simulink model "PID_enable_ROS2020b"  (R2020b)
settings: Solver=FixedStepAuto  StartTime=0.0  StopTime=inf  FixedStep=1/120  RelTol=1e-3
undefined symbols (not defined in the file): DiscIntNeverNeededParam, Flm, Frm, Jx_ref, Jy_ref, Jz_ref, m_ref, pos_ref, psi_ref, psidot_ref, Rlm, Rrm, t_ref, vel_ref, Yaw
libraries: robotlib x3, simulink x2, dspfdesign x1, aerolibanimutils x1
settings Model: Creator=iris  LastModifiedBy=iris
settings OptimizationCC: EnhancedBackFolding=on  PassReuseOutputArgsAs=Individual arguments  ZeroExternalMemoryAtStartup=off  ZeroInternalMemoryAtStartup=off  MaxStackSize=64  OptimizeBlockOrder=speed  DifferentSizesBufferReuse=on  OptimizationCustomize=off  EfficientTunableParamExpr=on
settings DebuggingCC: ParameterTunabilityLossMsg=error  SFMachineParentedDataDiag=error
settings HardwareCC: ProdBitPerPointer=32  ProdBitPerSizeT=32  ProdBitPerPtrDiffT=32  ProdLargestAtomicFloat=None  ProdIntDivRoundTo=Undefined  ProdEndianess=Unspecified  ProdWordSize=32  ProdHWDeviceType=Generic->Unspecified (assume 32-bit Generic)
settings SFSimCC: MATLABDynamicMemAlloc=off  SimTargetLang=C++
settings RTWCC: Description=Embedded Coder  SystemTargetFile=ert.tlc  HardwareBoard=Robot Operating System (ROS)  TLCOptions="-aInlineSetEventsForThisBaseRateFcn=TLC_FALSE -aSuppressMultiTaskScheduler=TLC_FALSE  -aRateBasedStepFcn=0"  TemplateMakefile=ert_default_tmf  Toolchain=Catkin  TargetLang=C++
settings CodeAppCC: ForceParamTrailComments=on  IgnoreCustomStorageClasses=off  OperatorAnnotations=on  SimulinkDataObjDesc=on  SFDataObjDesc=on  InsertBlockDesc=on
settings ERTTargetCC: SupportVariableSizeSignals=on

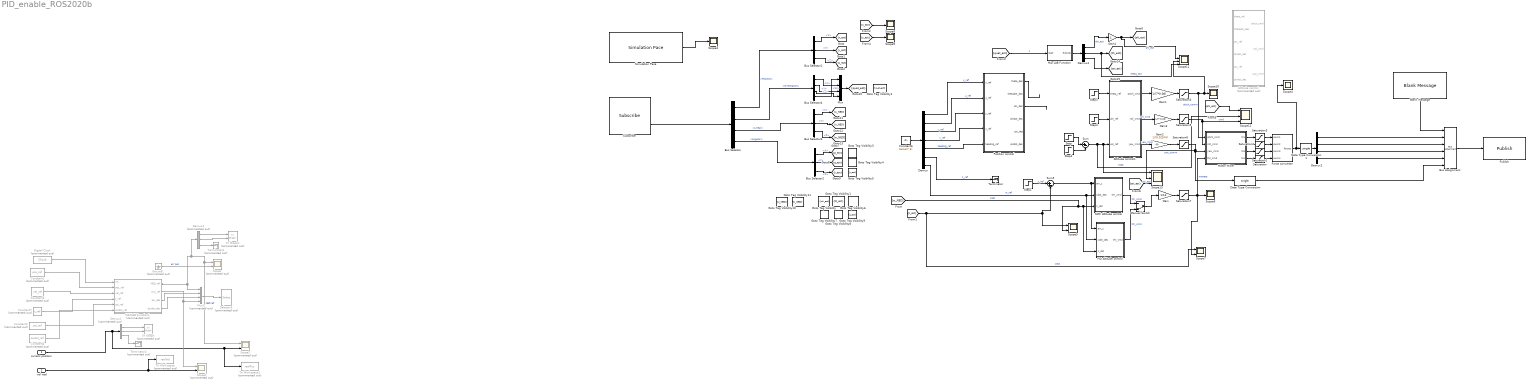
== system PID_enable_ROS2020b ==
  current position : Inport
  vel ned : Inport  Port=2
  Attitude control : Subsystem  Commented=on
  Attitude control1 : Subsystem
  Blank Message : robotlib/Blank Message  messageClass=Message  entityType=robotics_demo/QuadForce  messageType=robotics_demo/QuadForce  SampleTime=inf  legacyBusStruct=off
  Bus Assignment : BusAssignment  AssignedSignals=Frm,Rlm,Flm,Rrm,Yaw
  Bus Selector : BusSelector  OutputSignals=Pose.Pose.Position,Pose.Pose.Orientation,Twist.Twist.Linear,Twist.Twist.Angular
  Bus Selector1 : BusSelector  OutputSignals=X,Y,Z
  Bus Selector2 : BusSelector  OutputSignals=X,Y,Z
  Bus Selector3 : BusSelector  OutputSignals=X,Y,Z
  Bus Selector4 : BusSelector  OutputSignals=X,Y,Z,W
  Constant1 : Constant  Commented=on  Value=pos_ref
  Constant2 : Constant  Commented=on  Value=psi_ref
  Constant3 : Constant  Commented=on  Value=vel_ref
  Constant4 : Constant  Commented=on  Value=psidot_ref
  Constant5 : Constant  Commented=on  Value=t_ref
  Constant6 : Constant  Value=zeros(7,1)
  Data Type Conversion : DataTypeConversion  OutDataTypeStr=single
  Data Type Conversion1 : DataTypeConversion  OutDataTypeStr=single
  Demux : Demux  Outputs=7
  Demux1 : Demux  Commented=on  Outputs=3
  Demux2 : Demux
  Demux3 : Demux  Commented=on  Outputs=3
  Demux4 : Demux  Outputs=3
  Digital Clock : DigitalClock  Commented=on  SampleTime=-1
  Force converter : MATLAB Function  TreatAsAtomicUnit=on
  Gain : Gain  Gain=1/14
  Gain1 : Gain  Gain=1/(7*0.08)
  Gain2 : Gain  Gain=1/(0.025*4)
  Gain3 : Gain  Gain=1/(7*0.08)
  Gain4 : Gain
  Goto Tag Visibility : GotoTagVisibility  GotoTag=phi_est
  Goto Tag Visibility1 : GotoTagVisibility  GotoTag=th_est
  Goto Tag Visibility10 : GotoTagVisibility  GotoTag=u_NED
  Goto Tag Visibility11 : GotoTagVisibility  GotoTag=v_NED
  Goto Tag Visibility2 : GotoTagVisibility  GotoTag=quat_est
  Goto Tag Visibility3 : GotoTagVisibility  GotoTag=p_est
  Goto Tag Visibility4 : GotoTagVisibility  GotoTag=q_est
  Goto Tag Visibility5 : GotoTagVisibility  GotoTag=r_est
  Goto Tag Visibility6 : GotoTagVisibility  GotoTag=psi_est
  Goto Tag Visibility7 : GotoTagVisibility  GotoTag=x_est
  Goto Tag Visibility8 : GotoTagVisibility  GotoTag=y_est
  Goto Tag Visibility9 : GotoTagVisibility  GotoTag=z_est
  Ground1 : Ground  Commented=on
  MATLAB Function : MATLAB Function  TreatAsAtomicUnit=on
  MATLAB Function1 : MATLAB Function  Commented=on  TreatAsAtomicUnit=on
  Manual Switch : ManualSwitch  CurrentSetting=0
  Motor Mixer : MATLAB Function  TreatAsAtomicUnit=on
  Mux : Mux
  Mux1 : Mux  Commented=on
  PID Altitude control : Subsystem
  Position control : Subsystem
  Publish : robotlib/Publish  topicSource=Specify your own  topic=/motorForce  messageType=robotics_demo/QuadForce  legacyBusStruct=off  messageQueueLength=1
  SMC Altitude control : Subsystem
  Saturation : Saturate  UpperLimit=2000  LowerLimit=0
  Saturation1 : Saturate  UpperLimit=2000  LowerLimit=0
  Saturation2 : Saturate  UpperLimit=2000  LowerLimit=0
  Saturation3 : Saturate  UpperLimit=2000  LowerLimit=1000
  Saturation4 : Saturate  UpperLimit=1  LowerLimit=-1
  Saturation5 : Saturate  UpperLimit=1  LowerLimit=-1
  Saturation6 : Saturate  UpperLimit=1  LowerLimit=-1
  Saturation7 : Saturate  UpperLimit=1  LowerLimit=0
  Scope : Scope  Commented=on  NumInputPorts=2
  Scope1 : Scope  Commented=on  NumInputPorts=2
  Scope{3..4,6,8..10} (6 alike) : Scope
  Scope11 : Scope  NumInputPorts=4
  Scope12 : Scope  NumInputPorts=3
  Scope13 : Scope  NumInputPorts=3
  Scope2 : Scope  Commented=on  NumInputPorts=2
  Scope5 : Scope  NumInputPorts=2
  Scope7 : Scope  NumInputPorts=2
  Selector3 : Selector  Commented=on  InputPortWidth=8  IndexOptions=Index vector (dialog)  Indices=[1 6 2 7 4 3 8]  OutputSizes=1
  Simulation Pace : aerolibanimutils/Simulation Pace  SimulationPace=1  SleepMode=Auto  OutputPaceError=on  SampleTime=1/30
  Step : Step  Time=6  After=10/180*pi  SampleTime=0
  Step1 : Step  After=10
  Step2 : Step  Time=7  After=10/180*pi  SampleTime=0
  Step3 : Step  Time=0  After=0  SampleTime=0
  Step4 : Step  Time=0  After=0  SampleTime=0
  Subscribe : robotlib/Subscribe  topicSource=Specify your own  topic=/odom  messageType=nav_msgs/Odometry  SampleTime=-1  legacyBusStruct=off  messageQueueLength=1
  Sum : Sum  Inputs=|+-
  Sum5 : Sum  Inputs=|+-
  Terminator : Terminator
  Terminator2 : Terminator  Commented=on
  Terminator3 : Terminator  Commented=on
  To Workspace : ToWorkspace  Commented=on  VariableName=realVel  SaveFormat=Timeseries  SampleTime=-1
  To Workspace1 : ToWorkspace  Commented=on  VariableName=realPos  SaveFormat=Timeseries  SampleTime=-1
  XY Graph : simulink/Sinks/XY Graph  Commented=on  xmin=-20  xmax=20  ymin=-20  ymax=20  st=-1
  XY Graph1 : simulink/Sinks/XY Graph  Commented=on  xmin=-20  xmax=20  ymin=-20  ymax=20  st=-1
  tag scope: p_est=scoped, phi_est=scoped, psi_est=scoped, q_est=scoped, quat_est=scoped, r_est=scoped, th_est=scoped, u_NED=scoped, v_NED=scoped, x_est=scoped, y_est=scoped, z_est=scoped
  wires:
  Demux1/1 -> XY Graph/1
  current position/1 -> To Workspace1/1, Scope2/2, Demux1/1
  Demux3/3 -> Terminator3/1
  Demux3/2 -> XY Graph1/2
  Constant2/1 -> MATLAB Function1/5(psi_ref)
  MATLAB Function1/3(psi_des) -> Mux1/2
  Demux1/2 -> XY Graph/2
  Mux1/1 -> Selector3/1
  Constant3/1 -> MATLAB Function1/3(vel_ref)
  MATLAB Function1/2(uvw_ref) -> Scope1/1, Mux1/4
  Constant1/1 -> MATLAB Function1/2(pos_ref)
  Ground1/1 -> Scope/2  "err pos"
  vel ned/1 -> To Workspace/1, Scope1/2
  MATLAB Function1/1(NED_ref) -> Mux1/1, Demux3/1, Scope2/1, Scope/1  "NED ref"
  Constant5/1 -> MATLAB Function1/4(t_ref)
  Demux3/1 -> XY Graph1/1
  Digital Clock/1 -> MATLAB Function1/1(clk)
  MATLAB Function1/4(psidot_des) -> Mux1/3
  Demux1/3 -> Terminator2/1
  Constant4/1 -> MATLAB Function1/6(psidot_ref)
  Motor Mixer/3(M3) -> Saturation1/1
  Demux4/1 -> Gain4/1  "phi_est"
  SMC Altitude control/1(thr_cmd) -> Manual Switch/1  "thr_cmd"
  Demux4/2 -> [th_est], Scope11/4  "theta_est"
  Saturation2/1 -> Force converter/2(pwm2)
  Bus Selector/1 -> Bus Selector1/1  "<Position>"
  Bus Selector3/1 -> [u_NED]  "<X>"
  Demux/6 -> Terminator/1  "z_ref"
  Demux/7 -> PID Altitude control/2(zdot_des), SMC Altitude control/2(zdot_des)  "w_ref"
  Demux/2 -> Position control/2(u_ref)  "u_ref"
  Saturation/1 -> Force converter/4(pwm4)
  PID Altitude control/1(thr_cmd) -> Manual Switch/2  "thr_cmd"
  Bus Selector/2 -> Bus Selector4/1  "<Orientation>"
  Attitude control1/1(pitch_cmd) -> Gain1/1
  Bus Selector2/3 -> [r_est]  "<Z>"
  [w_NED] -> PID Altitude control/3(z_dot), SMC Altitude control/3(z_dot), Scope5/2  "zdot"
  Gain1/1 -> Saturation4/1
  [quat_est] -> MATLAB Function/1(quat)  "z"
  Demux/5 -> Position control/5(heading_ref)  "heading_ref"
  Gain3/1 -> Saturation5/1
  Demux/3 -> Position control/3(y_ref)  "y_ref"
  Bus Selector1/3 -> [z_est]  "<Z>"
  Saturation3/1 -> Force converter/1(pwm1)
  Subscribe/2 -> Bus Selector/1
  Gain/1 -> Saturation7/1
  Sum5/1 -> PID Altitude control/1(err_z), SMC Altitude control/1(err_z)
  Bus Selector4/2 -> Mux/3  "<Y>"
  Manual Switch/1 -> Gain/1
  Bus Selector4/3 -> Mux/4  "<Z>"
  Motor Mixer/1(M1) -> Saturation3/1
  Bus Selector/4 -> Bus Selector2/1  "<Angular>"
  Bus Selector3/3 -> [w_NED]  "<Z>"
  Gain2/1 -> Saturation6/1
  Constant6/1 -> Demux/1
  Bus Selector4/1 -> Mux/2  "<X>"
  Bus Assignment/1 -> Publish/1
  Mux/1 -> [quat_est]
  Blank Message/1 -> Bus Assignment/1
  Force converter/1(forces) -> Scope4/1, Data Type Conversion1/1
  Saturation1/1 -> Force converter/3(pwm3)
  Attitude control1/2(roll_cmd) -> Gain3/1  "roll_cmd"
  Bus Selector2/1 -> [p_est]  "<X>"
  Attitude control1/3(yaw_cmd) -> Gain2/1  "yaw_cmd"
  Step1/1 -> Sum5/1  "z_ref"
  Saturation7/1 -> Scope7/2, Motor Mixer/4(thr_cmd), Scope6/1  "maneta"
  Bus Selector1/2 -> [y_est]  "<Y>"
  Data Type Conversion/1 -> Bus Assignment/6
  Demux4/3 -> [psi_est]
  MATLAB Function/1(eulAng) -> Demux4/1
  Bus Selector/3 -> Bus Selector3/1  "<Linear>"
  Data Type Conversion1/1 -> Demux2/1
  Bus Selector1/1 -> [x_est]  "<X>"
  [z_est] -> Scope7/1, Scope5/1, Sum5/2  "zest"
  Motor Mixer/2(M2) -> Saturation2/1
  Bus Selector2/2 -> [q_est]  "<Y>"
  Demux/4 -> Position control/4(v_ref)  "v_ref"
  Demux/1 -> Position control/1(x_ref)  "x_ref"
  Saturation4/1 -> Motor Mixer/1(pitch_cmd), Scope11/3, Scope10/1  "pitch_comm"
  Motor Mixer/4(M4) -> Saturation/1
  Bus Selector3/2 -> [v_NED]  "<Y>"
  Simulation Pace/1 -> Scope3/1
  Step/1 -> Sum/1
  Sum/1 -> Attitude control1/3(psi_ref), Scope13/1, Scope12/2  "step"
  Step2/1 -> Sum/2
  [y_est] -> Scope9/1
  [x_est] -> Scope8/1
  Saturation5/1 -> Motor Mixer/2(roll_cmd), Scope12/3  "cmd"
  Demux2/1 -> Bus Assignment/2
  Demux2/2 -> Bus Assignment/3
  Demux2/4 -> Bus Assignment/5
  Demux2/3 -> Bus Assignment/4
  Bus Selector4/4 -> Mux/1  "<W>"
  Gain4/1 -> [phi_est], Scope11/2  "phi_est"
  [phi_est] -> Scope12/1
  Saturation6/1 -> Scope13/2, Data Type Conversion/1, Motor Mixer/3(yaw_cmd)  "yaw_comm"
  [psi_est] -> Scope13/3  "psi_est"
  Position control/1(theta_des) -> ?
  Position control/3(phi_des) -> ?
  Step3/1 -> Attitude control1/1(theta_ref)
  Step4/1 -> Attitude control1/2(phi_ref)

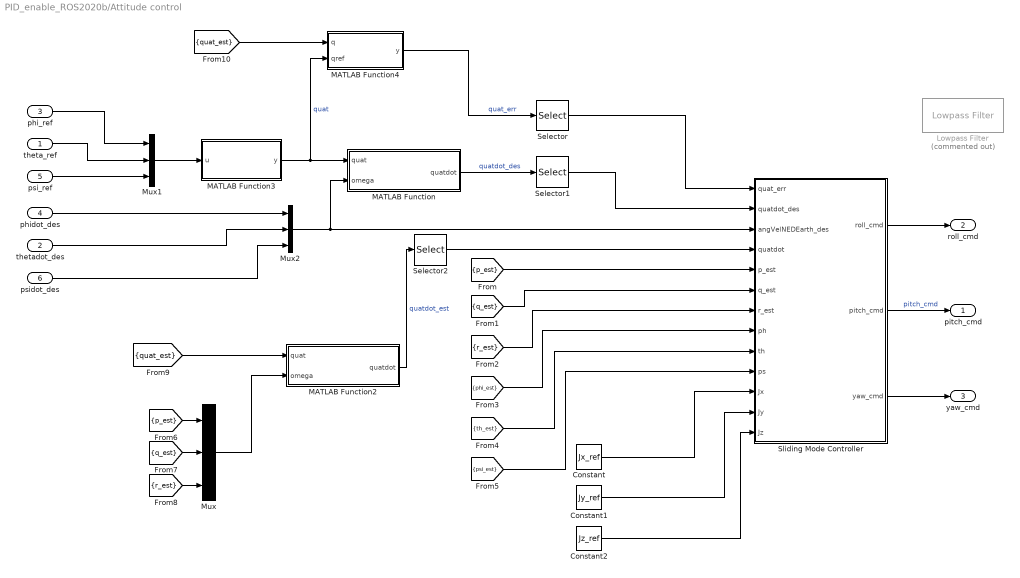
== system PID_enable_ROS2020b/Attitude control ==
  theta_ref : Inport
  thetadot_des : Inport  Port=2
  phi_ref : Inport  Port=3
  phidot_des : Inport  Port=4
  psi_ref : Inport  Port=5
  psidot_des : Inport  Port=6
  Constant : Constant  Value=Jx_ref
  Constant1 : Constant  Value=Jy_ref
  Constant2 : Constant  Value=Jz_ref
  Lowpass Filter : dspfdesign/Lowpass Filter  Commented=on  FilterType=FIR  DesignForMinimumOrder=on  FilterOrder=50  PassbandFrequency=100  StopbandFrequency=1000  PassbandRipple=0.1  StopbandAttenuation=40  InheritSampleRate=off  SampleRate=44100  SimulateUsing=Interpreted execution  roundingMode=Floor  coeffsDataTypeStr=fixdt(1,16)
  MATLAB Function : MATLAB Function  TreatAsAtomicUnit=on
  MATLAB Function2 : MATLAB Function  TreatAsAtomicUnit=on
  MATLAB Function3 : MATLAB Function  TreatAsAtomicUnit=on
  MATLAB Function4 : MATLAB Function  TreatAsAtomicUnit=on
  Mux : Mux  Inputs=3
  Mux1 : Mux  Inputs=3
  Mux2 : Mux  Inputs=3
  Selector : Selector  InputPortWidth=4  IndexOptions=Index vector (dialog)  Indices=[2:4]  OutputSizes=1
  Selector1 : Selector  InputPortWidth=4  IndexOptions=Index vector (dialog)  Indices=[2:4]  OutputSizes=1
  Selector2 : Selector  InputPortWidth=4  IndexOptions=Index vector (dialog)  Indices=[2:4]  OutputSizes=1
  Sliding Mode Controller : MATLAB Function  TreatAsAtomicUnit=on
  pitch_cmd : Outport  VectorParamsAs1DForOutWhenUnconnected=off
  roll_cmd : Outport  Port=2  VectorParamsAs1DForOutWhenUnconnected=off
  yaw_cmd : Outport  Port=3  VectorParamsAs1DForOutWhenUnconnected=off
  wires:
  [quat_est] -> MATLAB Function2/1(quat)
  MATLAB Function4/1(y) -> Selector/1  "quat_err"
  Mux1/1 -> MATLAB Function3/1(u)
  [r_est] -> Mux/3
  thetadot_des/1 -> Mux2/2
  [phi_est] -> Sliding Mode Controller/8(ph)
  [q_est] -> Mux/2
  Selector1/1 -> Sliding Mode Controller/2(quatdot_des)
  MATLAB Function2/1(quatdot) -> Selector2/1  "quatdot_est"
  [psi_est] -> Sliding Mode Controller/10(ps)
  Mux2/1 -> MATLAB Function/2(omega), Sliding Mode Controller/3(angVelNEDEarth_des)
  Selector/1 -> Sliding Mode Controller/1(quat_err)
  MATLAB Function/1(quatdot) -> Selector1/1  "quatdot_des"
  Mux/1 -> MATLAB Function2/2(omega)
  [q_est] -> Sliding Mode Controller/6(q_est)
  MATLAB Function3/1(y) -> MATLAB Function4/2(qref), MATLAB Function/1(quat)  "quat"
  [p_est] -> Sliding Mode Controller/5(p_est)
  Constant2/1 -> Sliding Mode Controller/13(Jz)
  Constant1/1 -> Sliding Mode Controller/12(Jy)
  [r_est] -> Sliding Mode Controller/7(r_est)
  Selector2/1 -> Sliding Mode Controller/4(quatdot)
  [th_est] -> Sliding Mode Controller/9(th)
  [p_est] -> Mux/1
  Sliding Mode Controller/2(pitch_cmd) -> pitch_cmd/1  "pitch_cmd"
  Constant/1 -> Sliding Mode Controller/11(Jx)
  theta_ref/1 -> Mux1/2
  phi_ref/1 -> Mux1/1
  psi_ref/1 -> Mux1/3
  [quat_est] -> MATLAB Function4/1(q)
  phidot_des/1 -> Mux2/1
  psidot_des/1 -> Mux2/3
  Sliding Mode Controller/1(roll_cmd) -> roll_cmd/1
  Sliding Mode Controller/3(yaw_cmd) -> yaw_cmd/1

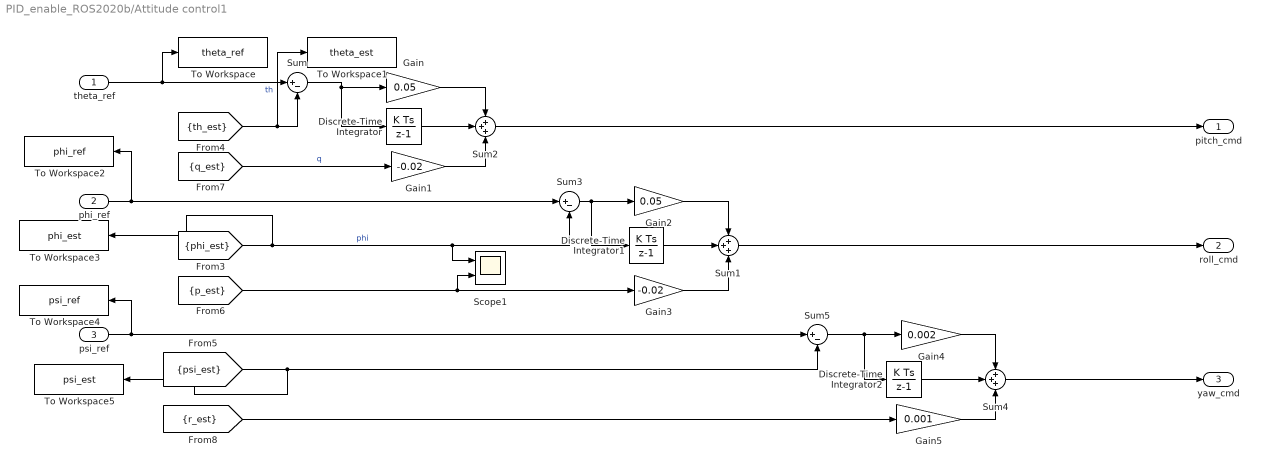
== system PID_enable_ROS2020b/Attitude control1 ==
  theta_ref : Inport
  phi_ref : Inport  Port=2
  psi_ref : Inport  Port=3
  Discrete-Time Integrator : DiscreteIntegrator  gainval=0.001  SampleTime=-1  ICPrevOutput=DiscIntNeverNeededParam  ICPrevScaledInput=DiscIntNeverNeededParam
  Discrete-Time Integrator1 : DiscreteIntegrator  gainval=0.001  SampleTime=-1  ICPrevOutput=DiscIntNeverNeededParam  ICPrevScaledInput=DiscIntNeverNeededParam
  Discrete-Time Integrator2 : DiscreteIntegrator  gainval=0.001  SampleTime=-1  UpperSaturationLimit=0.2  LowerSaturationLimit=-0.2  ICPrevOutput=DiscIntNeverNeededParam  ICPrevScaledInput=DiscIntNeverNeededParam
  Gain : Gain  Gain=0.05
  Gain1 : Gain  Gain=-0.02
  Gain2 : Gain  Gain=0.05
  Gain3 : Gain  Gain=-0.02
  Gain4 : Gain  Gain=0.002
  Gain5 : Gain  Gain=0.001
  Scope1 : Scope  NumInputPorts=2
  Sum : Sum  Inputs=|+-
  Sum1 : Sum  Inputs=+++
  Sum2 : Sum  Inputs=+++
  Sum3 : Sum  Inputs=|+-
  Sum4 : Sum  Inputs=+++
  Sum5 : Sum  Inputs=|+-
  To Workspace : ToWorkspace  VariableName=theta_ref  SampleTime=-1
      settings: Save2DSignal=2-D array (concatenate along first dimension)
  To Workspace1 : ToWorkspace  VariableName=theta_est  SampleTime=-1
      settings: Save2DSignal=2-D array (concatenate along first dimension)
  To Workspace2 : ToWorkspace  VariableName=phi_ref  SampleTime=-1
      settings: Save2DSignal=2-D array (concatenate along first dimension)
  To Workspace3 : ToWorkspace  VariableName=phi_est  SampleTime=-1
      settings: Save2DSignal=2-D array (concatenate along first dimension)
  To Workspace4 : ToWorkspace  VariableName=psi_ref  SampleTime=-1
      settings: Save2DSignal=2-D array (concatenate along first dimension)
  To Workspace5 : ToWorkspace  VariableName=psi_est  SampleTime=-1
      settings: Save2DSignal=2-D array (concatenate along first dimension)
  pitch_cmd : Outport  VectorParamsAs1DForOutWhenUnconnected=off
  roll_cmd : Outport  Port=2  VectorParamsAs1DForOutWhenUnconnected=off
  yaw_cmd : Outport  Port=3  VectorParamsAs1DForOutWhenUnconnected=off
  wires:
  [phi_est] -> To Workspace3/1, Scope1/1, Sum3/2  "phi"
  [psi_est] -> To Workspace5/1, Sum5/2
  [th_est] -> To Workspace1/1, Sum/2  "th"
  Sum2/1 -> pitch_cmd/1
  phi_ref/1 -> To Workspace2/1, Sum3/1
  psi_ref/1 -> To Workspace4/1, Sum5/1
  Sum1/1 -> roll_cmd/1
  Sum4/1 -> yaw_cmd/1
  [q_est] -> Gain1/1  "q"
  Discrete-Time Integrator/1 -> Sum2/2
  Gain/1 -> Sum2/1
  Gain1/1 -> Sum2/3
  Discrete-Time Integrator1/1 -> Sum1/2
  Sum3/1 -> Discrete-Time Integrator1/1, Gain2/1
  Gain2/1 -> Sum1/1
  Gain3/1 -> Sum1/3
  [p_est] -> Scope1/2, Gain3/1
  Sum/1 -> Discrete-Time Integrator/1, Gain/1
  theta_ref/1 -> To Workspace/1, Sum/1
  Gain5/1 -> Sum4/3
  Gain4/1 -> Sum4/1
  Sum5/1 -> Discrete-Time Integrator2/1, Gain4/1
  Discrete-Time Integrator2/1 -> Sum4/2
  [r_est] -> Gain5/1

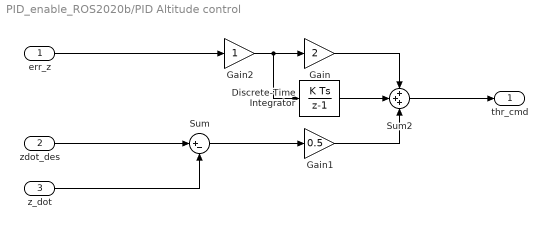
== system PID_enable_ROS2020b/PID Altitude control ==
  err_z : Inport
  zdot_des : Inport  Port=2
  z_dot : Inport  Port=3
  Discrete-Time Integrator : DiscreteIntegrator  gainval=0.7  SampleTime=-1  ICPrevOutput=DiscIntNeverNeededParam  ICPrevScaledInput=DiscIntNeverNeededParam
  Gain : Gain  Gain=2
  Gain1 : Gain  Gain=0.5
  Gain2 : Gain
  Sum : Sum  Inputs=|+-
  Sum2 : Sum  Inputs=+++
  thr_cmd : Outport  VectorParamsAs1DForOutWhenUnconnected=off
  wires:
  Sum2/1 -> thr_cmd/1
  zdot_des/1 -> Sum/1
  Gain/1 -> Sum2/1
  err_z/1 -> Gain2/1
  Gain1/1 -> Sum2/3
  Discrete-Time Integrator/1 -> Sum2/2
  Gain2/1 -> Discrete-Time Integrator/1, Gain/1
  z_dot/1 -> Sum/2
  Sum/1 -> Gain1/1

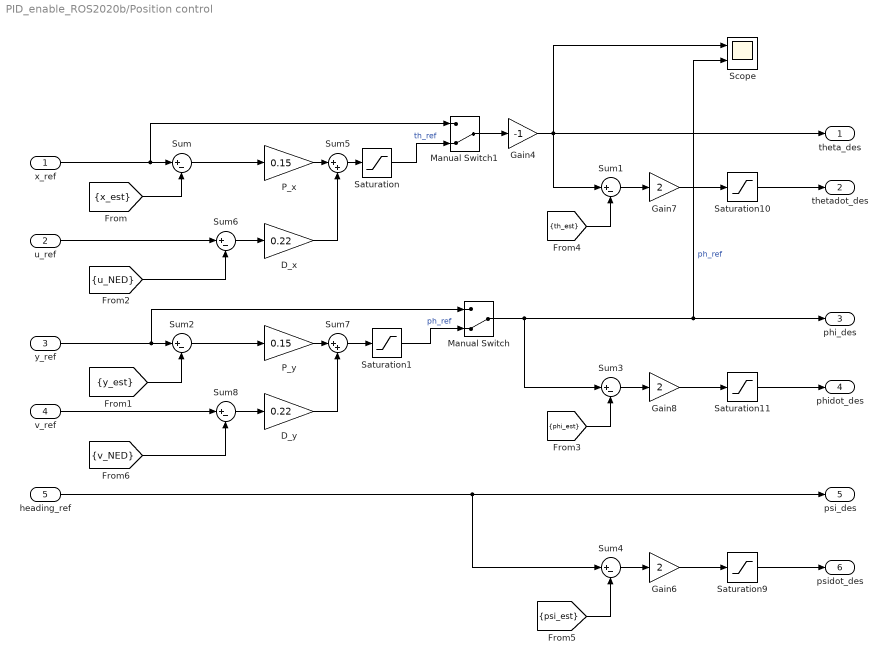
== system PID_enable_ROS2020b/Position control ==
  x_ref : Inport
  u_ref : Inport  Port=2
  y_ref : Inport  Port=3
  v_ref : Inport  Port=4
  heading_ref : Inport  Port=5
  D_x : Gain  Gain=0.22
  D_y : Gain  Gain=0.22
  Gain4 : Gain  Gain=-1
  Gain6 : Gain  Gain=2
  Gain7 : Gain  Gain=2
  Gain8 : Gain  Gain=2
  Manual Switch : ManualSwitch  CurrentSetting=0
  Manual Switch1 : ManualSwitch  CurrentSetting=0
  P_x : Gain  Gain=0.15
  P_y : Gain  Gain=0.15
  Saturation : Saturate  UpperLimit=30/180*pi  LowerLimit=-30/180*pi
  Saturation1 : Saturate  UpperLimit=30/180*pi  LowerLimit=-30/180*pi
  Saturation10 : Saturate  UpperLimit=1  LowerLimit=-1
  Saturation11 : Saturate  UpperLimit=1  LowerLimit=-1
  Saturation9 : Saturate
  Scope : Scope  NumInputPorts=2
  Sum{,1..4,6,8} (7 alike) : Sum  Inputs=|+-
  Sum5 : Sum  Inputs=|++
  Sum7 : Sum  Inputs=|++
  theta_des : Outport  VectorParamsAs1DForOutWhenUnconnected=off
  thetadot_des : Outport  Port=2  VectorParamsAs1DForOutWhenUnconnected=off
  phi_des : Outport  Port=3  VectorParamsAs1DForOutWhenUnconnected=off
  phidot_des : Outport  Port=4  VectorParamsAs1DForOutWhenUnconnected=off
  psi_des : Outport  Port=5  VectorParamsAs1DForOutWhenUnconnected=off
  psidot_des : Outport  Port=6  VectorParamsAs1DForOutWhenUnconnected=off
  wires:
  Manual Switch/1 -> phi_des/1, Scope/2, Sum3/1  "ph_ref"
  y_ref/1 -> Manual Switch/1, Sum2/1
  Sum1/1 -> Gain7/1
  [x_est] -> Sum/2
  [y_est] -> Sum2/2
  Saturation9/1 -> psidot_des/1
  Saturation1/1 -> Manual Switch/2  "ph_ref"
  Gain4/1 -> Sum1/1, theta_des/1, Scope/1
  Saturation/1 -> Manual Switch1/2  "th_ref"
  heading_ref/1 -> psi_des/1, Sum4/1
  Sum2/1 -> P_y/1
  x_ref/1 -> Manual Switch1/1, Sum/1
  Sum/1 -> P_x/1
  [psi_est] -> Sum4/2
  [phi_est] -> Sum3/2
  Gain6/1 -> Saturation9/1
  Manual Switch1/1 -> Gain4/1
  Sum4/1 -> Gain6/1
  Gain7/1 -> Saturation10/1
  Sum3/1 -> Gain8/1
  Gain8/1 -> Saturation11/1
  [th_est] -> Sum1/2
  Saturation10/1 -> thetadot_des/1
  Saturation11/1 -> phidot_des/1
  P_x/1 -> Sum5/1
  Sum5/1 -> Saturation/1
  D_x/1 -> Sum5/2
  Sum6/1 -> D_x/1
  u_ref/1 -> Sum6/1
  [u_NED] -> Sum6/2
  Sum7/1 -> Saturation1/1
  P_y/1 -> Sum7/1
  D_y/1 -> Sum7/2
  Sum8/1 -> D_y/1
  [v_NED] -> Sum8/2
  v_ref/1 -> Sum8/1

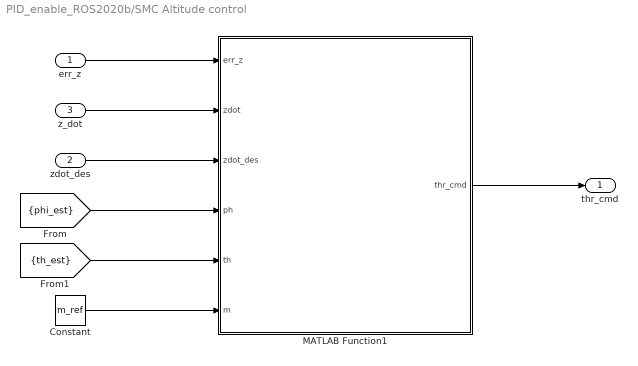
== system PID_enable_ROS2020b/SMC Altitude control ==
  err_z : Inport
  zdot_des : Inport  Port=2
  z_dot : Inport  Port=3
  Constant : Constant  Value=m_ref
  MATLAB Function1 : MATLAB Function  TreatAsAtomicUnit=on
  thr_cmd : Outport  VectorParamsAs1DForOutWhenUnconnected=off
  wires:
  MATLAB Function1/1(thr_cmd) -> thr_cmd/1
  z_dot/1 -> MATLAB Function1/2(zdot)
  err_z/1 -> MATLAB Function1/1(err_z)
  [phi_est] -> MATLAB Function1/4(ph)
  zdot_des/1 -> MATLAB Function1/3(zdot_des)
  [th_est] -> MATLAB Function1/5(th)
  Constant/1 -> MATLAB Function1/6(m)

== matlab function PID_enable_ROS2020b/Attitude control/MATLAB Function2 ==
  data: quat input; quatdot output; omega input
function quatdot = omega2quat(quat,omega)

p = omega(1);
q = omega(2);
r = omega(3);
Omega = [ 0, -p, -q, -r; p, 0, r, -q; q, -r, 0, p; r, q, -p, 0 ];
quatdot = 0.5*Omega*quat;

end

== matlab function PID_enable_ROS2020b/Attitude control/MATLAB Function3 ==
  data: u input; y output
function y = eulref2quatref(u)

y = eul2quat(u','XYZ')';

end

== matlab function PID_enable_ROS2020b/Attitude control/MATLAB Function4 ==
  data: y output; q input; qref input
function y =  errquat(q,qref)

y = quatprod([ q(1); -q(2:4) ]/norm(q), qref);

end

== matlab function PID_enable_ROS2020b/Attitude control/MATLAB Function ==
  data: quat input; quatdot output; omega input
function quatdot = omega2quat(quat,omega)

p = omega(1);
q = omega(2);
r = omega(3);
Omega = [ 0, -p, -q, -r; p, 0, r, -q; q, -r, 0, p; r, q, -p, 0 ];
quatdot = 0.5*Omega*quat;

end

== matlab function PID_enable_ROS2020b/Motor Mixer ==
  data: pitch_cmd input; M1 output; roll_cmd input; yaw_cmd input; thr_cmd input; M2 output; M3 output; M4 output
function [M1, M2, M3, M4] = motor_mixer(pitch_cmd, roll_cmd, yaw_cmd, thr_cmd)

idle = 1000;
% K_thr = 800;
% K_roll = 500;
% K_pitch = 500;
% K_yaw = 500;
% 
% % out = idle*ones(4,1) + K_thr*eye(4)*thr_cmd + K_roll*diag([-1, 1, 1, -1])*...
% %     roll_cmd + K_pitch*diag([1, -1, 1, -1])*pitch_cmd + ...
% %     K_yaw*diag([-1, -1, 1, 1])*yaw_cmd; % no matrix!
% 
% out = idle*ones(4,1) + K_thr*ones(4,1)*thr_cmd + K_roll*[-1, 1, 1, -1]'*...
%     roll_cmd + K_pitch*[1, -1, 1, -1]'*pitch_cmd + ...
%     K_yaw*[-1, -1, 1, 1]'*yaw_cmd; 
% 
% 
% 
% M1 = out(1);
% M2 = out(2);
% M3 = out(3);
% M4 = out(4);

M1 = (((-roll_cmd - pitch_cmd )/2*thr_cmd + thr_cmd)*1000 + idle);
M2 = (((roll_cmd + pitch_cmd)/2*thr_cmd + thr_cmd)*1000 + idle);
M3 = (((roll_cmd - pitch_cmd )/2*thr_cmd + thr_cmd)*1000 + idle);
M4 = (((-roll_cmd + pitch_cmd )/2*thr_cmd + thr_cmd)*1000 + idle);

end

== matlab function PID_enable_ROS2020b/MATLAB Function1 ==
  data: clk input; NED_ref output; uvw_ref output; psi_des output; pos_ref input; vel_ref input; t_ref input; psi_ref input; psidot_ref input; psidot_des output
function [ NED_ref, uvw_ref, psi_des, psidot_des]  = trajectoryPlanner(clk,pos_ref,vel_ref,t_ref, psi_ref, psidot_ref)

if clk <= t_ref(end)
    currTime = find(clk >= t_ref);
    NED_ref = pos_ref(currTime(end),:);
    uvw_ref = vel_ref(currTime(end),:);
    psi_des = psi_ref(currTime(end),:);
    psidot_des = psidot_ref(currTime(end),:);
else
    NED_ref = pos_ref(end,:);
    uvw_ref = vel_ref(end,:);
    psi_des = psi_ref(end,:);
    psidot_des = psidot_ref(end,:);
end

== matlab function PID_enable_ROS2020b/Force converter ==
  data: pwm1 input; forces output; pwm2 input; pwm3 input; pwm4 input
function forces = fcn(pwm1, pwm2, pwm3, pwm4)

% l = 0.2;
% P = [1.163247673946401e-05,-0.020227124498192,8.151335788071506];
% Q = [2.660432014565793e-07,-4.679737999801719e-04,0.204583957778948];
% u = zeros(6,1);
% u(3) = -(polyval(P,pwm1) + polyval(P,pwm2) + polyval(P,pwm3) + polyval(P,pwm4));
% u(4) = (polyval(P,pwm3) + polyval(P,pwm2) - polyval(P,pwm1) - polyval(P,pwm4))*l;
% u(5) = (polyval(P,pwm1) + polyval(P,pwm3) - polyval(P,pwm2) - polyval(P,pwm4))*l;
% u(6) = polyval(Q,pwm3) + polyval(Q,pwm4) - polyval(Q,pwm1) - polyval(Q,pwm2);
l = 0.1;
P = [2.381731e-6, -0.003628,1.177280];
Q = [2.660432014565793e-07,-4.679737999801719e-04,0.204583957778948];
u = zeros(6,1);
u(3) = -(polyval(P,pwm1) + polyval(P,pwm2) + polyval(P,pwm3) + polyval(P,pwm4));
u(4) = (polyval(P,pwm3) + polyval(P,pwm2) - polyval(P,pwm1) - polyval(P,pwm4))*l;
u(5) = (polyval(P,pwm1) + polyval(P,pwm3) - polyval(P,pwm2) - polyval(P,pwm4))*l;
u(6) = polyval(Q,pwm3) + polyval(Q,pwm4) - polyval(Q,pwm1) - polyval(Q,pwm2);

forces = zeros(4,1);
forces(1,1) = polyval(P,pwm1);
forces(2,1) = polyval(P,pwm2);
forces(3,1) = polyval(P,pwm3);
forces(4,1) = polyval(P,pwm4);

for i=1:4
    if forces(i,1) < 0
        forces(i,1) = 0;
    end

end

== matlab function PID_enable_ROS2020b/SMC Altitude control/MATLAB Function1 ==
  data: err_z input; thr_cmd output; zdot input; zdot_des input; ph input; th input; m input
function thr_cmd = ...
            thrustSMC(err_z,zdot,zdot_des,ph,th,m)

lamda = 100;     % 40
K = 15;          % 2
% Sliding surface
s = zdot_des - zdot + lamda*err_z;
% Command law (add zdotdot_des for traj plann)
% thr_cmd = -m/(cos(ph)*cos(th))*( -9.81 + 0 + lamda*(zdot_des - zdot))...
%          - K*sign(s);
% !! Changed the sign before 9.81 from + to - and it has less ss error!
thr_cmd = K*sign(s);
end

== matlab function PID_enable_ROS2020b/MATLAB Function ==
  data: quat input; eulAng output
function eulAng = quat2euler(quat)

% eulAng = quat2eul(quat','XYZ');
% Euler ZYX
phi = atan2(quat(3)*quat(4) + quat(1)*quat(2), 1/2 - (quat(2)^2 + quat(3)^2));
theta = asin(-2*(quat(2)*quat(4) - quat(1)*quat(3)));
psi = atan2(quat(2)*quat(3) + quat(1)*quat(4), 1/2 - (quat(3)^2 + quat(4)^2));

eulAng = [phi; theta; psi];

end

== matlab function PID_enable_ROS2020b/Attitude control/Sliding Mode Controller ==
  data: roll_cmd output; quat_err input; quatdot_des input; angVelNEDEarth_des input; quatdot input; p_est input; q_est input; pitch_cmd output; r_est input; ph input; th input; ps input; Jx input; Jy input; Jz input; yaw_cmd output
function [ roll_cmd, pitch_cmd, yaw_cmd ] = ...
        attitudeSMC(quat_err,quatdot_des,angVelNEDEarth_des,quatdot,...
        p_est,q_est,r_est,ph,th,ps,Jx,Jy,Jz)

phidot_des = angVelNEDEarth_des(1); 
thetadot_des = angVelNEDEarth_des(2);
psidot_des = angVelNEDEarth_des(3);
    
lamda = [ 20; 20; 10 ]; % 10   80 w/out "/cos(ps/2)" to psidot
K = [ -0.2; -0.2; -0.2 ]; % -0.05, -0.05, -0.25   -0.15 w/out "/cos(ps/2)" to psidot
phidot = p_est + tan(th)*(q_est*sin(ph) + r_est*cos(ph));
thetadot = q_est*cos(ph) - r_est*sin(ph);
psidot = (q_est*sin(ph) + r_est*cos(ph))/cos(th);

% Sliding surface
s = zeros(3,1);
s(1) = (phidot_des - phidot) + lamda(1)*(quat_err(1));
s(2) = (thetadot_des - thetadot) + lamda(2)*(quat_err(2));
s(3) = (psidot_des - psidot) + lamda(3)*(quat_err(3));

% Control law
roll_cmd = (Jx*(lamda(1)*(quatdot_des(1) - quatdot(1))/cos(ph*0)) - ...
        (Jy - Jz)*psidot*thetadot) - K(1)*sign(s(1));
pitch_cmd = (Jy*(lamda(2)*(quatdot_des(2) - quatdot(2))/cos(th*0)) - ...
        (Jz - Jx)*psidot*phidot) - K(2)*sign(s(2));
yaw_cmd = (Jz*(lamda(3)*(quatdot_des(3) - quatdot(3))/cos(0*ps/2)) - ...
        (Jx - Jy)*thetadot*phidot) - K(3)*sign(s(3));

end
